simulink model "inversor_multinivel_5_niveis"  (R2024a)
settings: Solver=VariableStepAuto  StartTime=0.0  StopTime=0.1  RelTol=1e-3
libraries: spsIGBTDiodeLib x24, spsDCVoltageSourceLib x6, simulink x6, spsCurrentMeasurementLib x3, spsVoltageMeasurementLib x3, spsThreePhaseParallelRLCBranchLib x1, spspowerguiLib x1
settings Model: Creator=victo  LastModifiedBy=victo

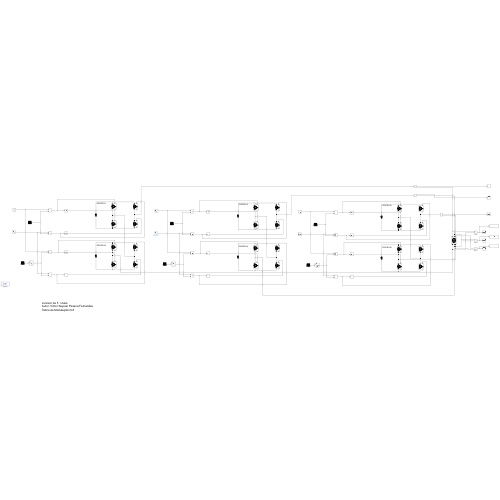
[thumbnail: Simulink's stored preview of the top-level diagram]
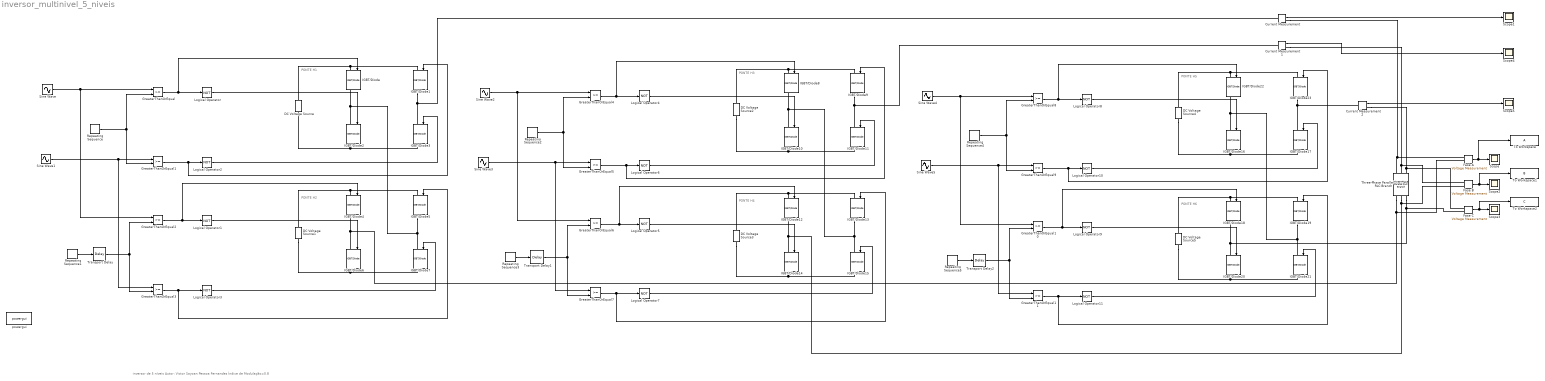
== system inversor_multinivel_5_niveis ==
  note: inversor de 5 níveis
      | Autor: Victor Sayoan Pessoa Fernandes
      | Índice de Modulação=0.8
  note: PONTE H1
  note: PONTE H2
  note: PONTE H3
  note: PONTE H4
  note: PONTE H6
  note: PONTE H5
  Current Measurement : spsCurrentMeasurementLib/Current Measurement  PhasorSimulation=off  OutputType=Complex  PSBequivalent=0
  Current Measurement1 : spsCurrentMeasurementLib/Current Measurement  PhasorSimulation=off  OutputType=Complex  PSBequivalent=0
  Current Measurement2 : spsCurrentMeasurementLib/Current Measurement  PhasorSimulation=off  OutputType=Complex  PSBequivalent=0
  DC Voltage Source{,1..5} (6 alike) : spsDCVoltageSourceLib/DC Voltage Source  Amplitude=160  Measurements=None
  Fase A : spsVoltageMeasurementLib/Voltage Measurement  PhasorSimulation=off  OutputType=Complex  PSBequivalent=0
  Fase B : spsVoltageMeasurementLib/Voltage Measurement  PhasorSimulation=off  OutputType=Complex  PSBequivalent=0
  Fase C : spsVoltageMeasurementLib/Voltage Measurement  PhasorSimulation=off  OutputType=Complex  PSBequivalent=0
  GreaterThanOrEqual{,1..11} (12 alike) : RelationalOperator  OutDataTypeStr=boolean  RndMeth=Simplest  InputSameDT=off
  IGBT/Diode{,1..23} (24 alike) : spsIGBTDiodeLib/IGBT//Diode  Ron=1e-3  Rs=1e5  Cs=inf  Measurements=on
  Logical Operator{,1..11} (12 alike) : Logic  Operator=NOT  AllPortsSameDT=off  OutDataTypeStr=boolean
  Repeating Sequence{,1..5} (6 alike) : simulink/Sources/Repeating Sequence  rep_seq_t=[0 0.5 1]/1000  rep_seq_y=[-1 1 -1]
  Scope{,1..5} (6 alike) : Scope
  Sine Wave : Sin  Frequency=2*pi*60  SampleTime=0
  Sine Wave1 : Sin  Amplitude=-1  Frequency=2*pi*60  SampleTime=0
  Sine Wave2 : Sin  Frequency=2*pi*60  Phase=(2*pi)/3  SampleTime=0
  Sine Wave3 : Sin  Amplitude=-1  Frequency=2*pi*60  Phase=(2*pi)/3  SampleTime=0
  Sine Wave4 : Sin  Frequency=2*pi*60  Phase=-(2*pi)/3  SampleTime=0
  Sine Wave5 : Sin  Amplitude=-1  Frequency=2*pi*60  Phase=-(2*pi)/3  SampleTime=0
  Three-Phase Parallel RLC Branch : spsThreePhaseParallelRLCBranchLib/Three-Phase Parallel RLC Branch  LConnTagsString=A|B|C  RConnTagsString=A|B|C  BranchType=RL  Resistance=1  Inductance=20e-3  Capacitance=1e-6  Measurements=None
  To Workspace : ToWorkspace  VariableName=A  SaveFormat=Structure With Time  SampleTime=-1
  To Workspace1 : ToWorkspace  VariableName=B  SaveFormat=Structure With Time  SampleTime=-1
  To Workspace2 : ToWorkspace  VariableName=C  SaveFormat=Structure With Time  SampleTime=-1
  Transport Delay : TransportDelay  DelayTime=0.3/1000
  Transport Delay1 : TransportDelay  DelayTime=0.3/1000
  Transport Delay2 : TransportDelay  DelayTime=0.3/1000
  powergui : spspowerguiLib/powergui  Priority=1  SimulationMode=Discrete  SampleTime=50e-6  frequency=60  Iterations=50  frequencyindice=0  Pbase=100e6  ErrMax=1e-4  UnitsV=kV  UnitsW=MW  buscounter=0  FunctionMessages=off  echomessages=off  EnableUseOfTLC=off  CurrentSourceSwitches=off  DisableSnubberDevices=off  DisableRonSwitches=off  DisableVfSwitches=off  DisplayEquations=off  AutomaticDiscreteSolvers=off  SolverType=Tustin/Backward Euler (TBE)  Interpol=off  ExternalGateDelay=off  methode=off  Ts=100  x0status=blocks  SPID=on  SwTol=0  HookPort=off  NonlinearTolerance=1e-4  nMaxIteration=100  ContinueOnMaxIteration=off  RestoreLinks=warning  ResistiveCurrentMeasurement=off  Frange=[0:2:500]  Ylog=off  Xlog=on  ShowGrid=off  save=off  variable=ZData  structure=0  ZoomFFT=off  StartTime=0.0  cycles=1  DisplayStyle=1  fundamental=60  FreqAxis=off  MaxFrequency=1000  frequencyindicesteady=1  RmsSteady=1  display=off
  wires:
  Logical Operator1/1 -> IGBT/Diode6/1
  Logical Operator2/1 -> IGBT/Diode3/1
  Logical Operator/1 -> IGBT/Diode2/1
  Logical Operator3/1 -> IGBT/Diode7/1
  GreaterThanOrEqual/1 -> IGBT/Diode/1, Logical Operator/1
  GreaterThanOrEqual1/1 -> Logical Operator2/1, IGBT/Diode1/1
  GreaterThanOrEqual2/1 -> IGBT/Diode4/1, Logical Operator1/1
  GreaterThanOrEqual3/1 -> IGBT/Diode5/1, Logical Operator3/1
  Repeating Sequence1/1 -> Transport Delay/1
  Repeating Sequence/1 -> GreaterThanOrEqual1/2, GreaterThanOrEqual/2
  Transport Delay/1 -> GreaterThanOrEqual2/2, GreaterThanOrEqual3/2
  Sine Wave1/1 -> GreaterThanOrEqual3/1, GreaterThanOrEqual1/1
  Sine Wave/1 -> GreaterThanOrEqual2/1, GreaterThanOrEqual/1
  Transport Delay1/1 -> GreaterThanOrEqual6/2, GreaterThanOrEqual7/2
  Repeating Sequence3/1 -> Transport Delay1/1
  Repeating Sequence2/1 -> GreaterThanOrEqual5/2, GreaterThanOrEqual4/2
  Logical Operator6/1 -> IGBT/Diode11/1
  Logical Operator5/1 -> IGBT/Diode14/1
  Sine Wave3/1 -> GreaterThanOrEqual7/1, GreaterThanOrEqual5/1
  Logical Operator4/1 -> IGBT/Diode10/1
  Logical Operator7/1 -> IGBT/Diode15/1
  GreaterThanOrEqual4/1 -> IGBT/Diode8/1, Logical Operator4/1
  GreaterThanOrEqual6/1 -> IGBT/Diode12/1, Logical Operator5/1
  GreaterThanOrEqual7/1 -> IGBT/Diode13/1, Logical Operator7/1
  GreaterThanOrEqual5/1 -> Logical Operator6/1, IGBT/Diode9/1
  Sine Wave2/1 -> GreaterThanOrEqual6/1, GreaterThanOrEqual4/1
  GreaterThanOrEqual8/1 -> IGBT/Diode22/1, Logical Operator8/1
  Logical Operator11/1 -> IGBT/Diode21/1
  GreaterThanOrEqual11/1 -> IGBT/Diode19/1, Logical Operator11/1
  Logical Operator8/1 -> IGBT/Diode16/1
  Logical Operator9/1 -> IGBT/Diode20/1
  Logical Operator10/1 -> IGBT/Diode17/1
  Repeating Sequence4/1 -> GreaterThanOrEqual9/2, GreaterThanOrEqual8/2
  Transport Delay2/1 -> GreaterThanOrEqual10/2, GreaterThanOrEqual11/2
  GreaterThanOrEqual10/1 -> IGBT/Diode18/1, Logical Operator9/1
  Repeating Sequence5/1 -> Transport Delay2/1
  Sine Wave5/1 -> GreaterThanOrEqual11/1, GreaterThanOrEqual9/1
  GreaterThanOrEqual9/1 -> Logical Operator10/1, IGBT/Diode23/1
  Sine Wave4/1 -> GreaterThanOrEqual10/1, GreaterThanOrEqual8/1
  Current Measurement/1 -> Scope1/1
  Current Measurement1/1 -> Scope4/1
  Current Measurement2/1 -> Scope5/1
  Fase A/1 -> To Workspace/1, Scope/1
  Fase C/1 -> To Workspace2/1, Scope3/1
  Fase B/1 -> To Workspace1/1, Scope2/1
  connections:
  IGBT/Diode/LConn1 -- IGBT/Diode1/LConn1 -- DC Voltage Source/RConn1
  IGBT/Diode3/RConn1 -- DC Voltage Source/LConn1 -- IGBT/Diode2/RConn1
  IGBT/Diode4/LConn1 -- IGBT/Diode5/LConn1 -- DC Voltage Source1/RConn1
  IGBT/Diode2/LConn1 -- IGBT/Diode/RConn1 -- IGBT/Diode7/LConn1 -- IGBT/Diode5/RConn1
  IGBT/Diode7/RConn1 -- DC Voltage Source1/LConn1 -- IGBT/Diode6/RConn1
  IGBT/Diode6/LConn1 -- Fase A/LConn2 -- Three-Phase Parallel RLC Branch/RConn1 -- IGBT/Diode4/RConn1
  IGBT/Diode12/LConn1 -- IGBT/Diode13/LConn1 -- DC Voltage Source3/RConn1
  IGBT/Diode8/LConn1 -- IGBT/Diode9/LConn1 -- DC Voltage Source2/RConn1
  IGBT/Diode10/RConn1 -- IGBT/Diode11/RConn1 -- DC Voltage Source2/LConn1
  IGBT/Diode13/RConn1 -- IGBT/Diode10/LConn1 -- IGBT/Diode8/RConn1 -- IGBT/Diode15/LConn1
  IGBT/Diode14/RConn1 -- IGBT/Diode15/RConn1 -- DC Voltage Source3/LConn1
  IGBT/Diode14/LConn1 -- Fase B/LConn2 -- Three-Phase Parallel RLC Branch/RConn2 -- IGBT/Diode12/RConn1
  IGBT/Diode20/RConn1 -- IGBT/Diode21/RConn1 -- DC Voltage Source5/LConn1
  IGBT/Diode16/RConn1 -- IGBT/Diode17/RConn1 -- DC Voltage Source4/LConn1
  IGBT/Diode20/LConn1 -- Fase C/LConn2 -- Three-Phase Parallel RLC Branch/RConn3 -- IGBT/Diode18/RConn1
  IGBT/Diode19/RConn1 -- IGBT/Diode21/LConn1 -- IGBT/Diode16/LConn1 -- IGBT/Diode22/RConn1
  IGBT/Diode22/LConn1 -- IGBT/Diode23/LConn1 -- DC Voltage Source4/RConn1
  IGBT/Diode18/LConn1 -- IGBT/Diode19/LConn1 -- DC Voltage Source5/RConn1
  Fase C/LConn1 -- Current Measurement2/RConn1 -- Three-Phase Parallel RLC Branch/LConn3
  IGBT/Diode9/RConn1 -- Current Measurement1/LConn1 -- IGBT/Diode11/LConn1
  IGBT/Diode1/RConn1 -- Current Measurement/LConn1 -- IGBT/Diode3/LConn1
  Fase A/LConn1 -- Current Measurement/RConn1 -- Three-Phase Parallel RLC Branch/LConn1
  Three-Phase Parallel RLC Branch/LConn2 -- Fase B/LConn1 -- Current Measurement1/RConn1
  IGBT/Diode23/RConn1 -- Current Measurement2/LConn1 -- IGBT/Diode17/LConn1
